simulink model "app_FaultMgr"  (R2016b)
settings: Solver=FixedStepDiscrete  StartTime=0.0  StopTime=10.0  FixedStep=0.001  RelTol=1e-3  EnableMultiTasking=on
PreLoadFcn:
  | try
  |    tapas_types('load');
  | catch
  |   disp('TAPAS WARNING: Tapas Types could not be loaded ...');
  | end
  | 
  | try
  |   app_types('load');
  | catch
  |   currdir =pwd;
  |   try
  |     cd('..\app_types\');
  |     app_types('load');
  |     cd(currdir);
  |   catch
  |     try
  |        cd('..\..\app_types\');
  |        app_types('load');
  |        cd(currdir);
  |     catch
  |        cd(currdir);
  |        disp('TAPAS WARNING: Application Types could not be loaded ...');
  |     end
  |   end
  |   try
  |       clear currdir;
  |   catch
  |      %Do nothing
  |   end
  | end
settings Model: Creator=kmansour  LastModifiedBy=Paul
settings DataIOCC: LimitDataPoints=on  SaveFormat=Array
settings OptimizationCC: LifeSpan=1
settings DebuggingCC: AllowSymbolicDim=off  SFUnexpectedBacktrackingDiag=warning  SFNoUnconditionalDefaultTransitionDiag=warning  SFExecutionAtInitializationDiag=none
settings HardwareCC: ProdBitPerPointer=32  ProdBitPerSizeT=32  ProdBitPerPtrDiffT=32  ProdLargestAtomicInteger=Long  ProdLargestAtomicFloat=Double  ProdWordSize=32  ProdHWDeviceType=Texas Instruments->TMS570 Cortex-R4
settings ModelReferenceCC: ModelReferenceNumInstancesAllowed=Single  PropagateSignalLabelsOutOfModel=off
settings RTWCC: SystemTargetFile=ert.tlc  GenCodeOnly=on  TemplateMakefile=ert_default_tmf  Description=Embedded Coder  GenerateReport=on  IncludeHyperlinkInReport=on  LaunchReport=on  GenerateTraceInfo=on  GenerateTraceReport=on  GenerateTraceReportSl=on  GenerateTraceReportSf=on  GenerateTraceReportEml=on
settings CodeAppCC: IgnoreCustomStorageClasses=off  MaxIdLength=63
settings ERTTargetCC: GenerateSampleERTMain=on  ERTSrcFileBannerTemplate=tapas_code_template.cgt  ERTHdrFileBannerTemplate=tapas_code_template.cgt  ERTDataSrcFileTemplate=tapas_code_template.cgt  ERTDataHdrFileTemplate=tapas_code_template.cgt  ERTCustomFileTemplate=example_file_process.tlc  ConvertIfToSwitch=off  SuppressUnreachableDefaultCases=off
settings ConfigComp: CovMetricSettings=dw  CovHtmlReporting=on  CovSaveCumulativeToWorkspaceVar=on  CovSaveSingleToWorkspaceVar=on  CovExternalEMLEnable=off

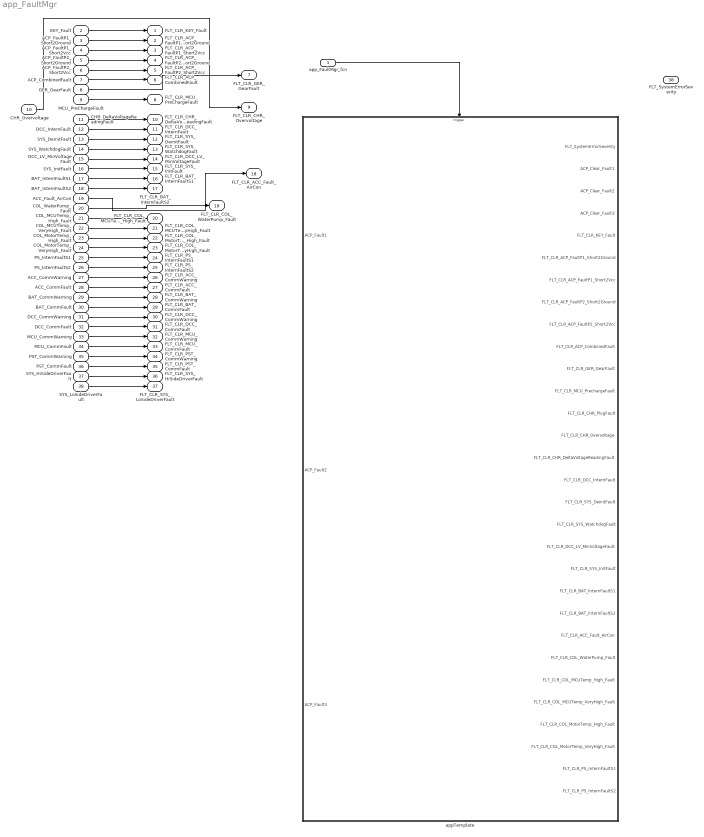
== system app_FaultMgr ==
  app_FaultMgr_fcn : Inport  SampleTime=1e-3  OutputFunctionCall=on
  KEY_Fault : Inport  Port=2
  ACP_FaultP1_Short2Ground : Inport  Port=3
  ACP_FaultP1_Short2Vcc : Inport  Port=4
  ACP_FaultP2_Short2Ground : Inport  Port=5
  ACP_FaultP2_Short2Vcc : Inport  Port=6
  ACP_CombinedFault : Inport  Port=7
  GER_GearFault : Inport  Port=8
  MCU_PreChargeFault : Inport  Port=9
  CHR_Overvoltage : Inport  Port=10
  CHR_DeltaVoltageReadingFault : Inport  Port=11
  DCC_InternFault : Inport  Port=12
  SYS_DeinitFault : Inport  Port=13
  SYS_WatchdogFault : Inport  Port=14
  DCC_LV_MinVoltageFault : Inport  Port=15
  SYS_InitFault : Inport  Port=16
  BAT_InternFaultS1 : Inport  Port=17
  BAT_InternFaultS2 : Inport  Port=18
  ACC_Fault_AirCon : Inport  Port=19
  COL_WaterPump_Fault : Inport  Port=20
  COL_MCUTemp_High_Fault : Inport  Port=21
  COL_MCUTemp_VeryHigh_Fault : Inport  Port=22
  COL_MotorTemp_High_Fault : Inport  Port=23
  COL_MotorTemp_VeryHigh_Fault : Inport  Port=24
  PS_InternFaultS1 : Inport  Port=25
  PS_InternFaultS2 : Inport  Port=26
  ACC_CommWarning : Inport  Port=27
  ACC_CommFault : Inport  Port=28
  BAT_CommWarning : Inport  Port=29
  BAT_CommFault : Inport  Port=30
  DCC_CommWarning : Inport  Port=31
  DCC_CommFault : Inport  Port=32
  MCU_CommWarning : Inport  Port=33
  MCU_CommFault : Inport  Port=34
  PST_CommWarning : Inport  Port=35
  PST_CommFault : Inport  Port=36
  SYS_HiSideDriverFault : Inport  Port=37
  SYS_LoSideDriverFault : Inport  Port=38
  appTemplate : Subsystem
  FLT_CLR_KEY_Fault : Outport
  FLT_CLR_ACP_FaultP1_Short2Ground : Outport  Port=2
  FLT_CLR_ACP_FaultP1_Short2Vcc : Outport  Port=3
  FLT_CLR_ACP_FaultP2_Short2Ground : Outport  Port=4
  FLT_CLR_ACP_FaultP2_Short2Vcc : Outport  Port=5
  FLT_CLR_ACP_CombinedFault : Outport  Port=6
  FLT_CLR_GER_GearFault : Outport  Port=7
  FLT_CLR_MCU_PreChargeFault : Outport  Port=8
  FLT_CLR_CHR_Overvoltage : Outport  Port=9
  FLT_CLR_CHR_DeltaVoltageReadingFault : Outport  Port=10
  FLT_CLR_DCC_InternFault : Outport  Port=11
  FLT_CLR_SYS_DeinitFault : Outport  Port=12
  FLT_CLR_SYS_WatchdogFault : Outport  Port=13
  FLT_CLR_DCC_LV_MinVoltageFault : Outport  Port=14
  FLT_CLR_SYS_InitFault : Outport  Port=15
  FLT_CLR_BAT_InternFaultS1 : Outport  Port=16
  FLT_CLR_BAT_InternFaultS2 : Outport  Port=17
  FLT_CLR_ACC_Fault_AirCon : Outport  Port=18
  FLT_CLR_COL_WaterPump_Fault : Outport  Port=19
  FLT_CLR_COL_MCUTemp_High_Fault : Outport  Port=20
  FLT_CLR_COL_MCUTemp_VeryHigh_Fault : Outport  Port=21
  FLT_CLR_COL_MotorTemp_High_Fault : Outport  Port=22
  FLT_CLR_COL_MotorTemp_VeryHigh_Fault : Outport  Port=23
  FLT_CLR_PS_InternFaultS1 : Outport  Port=24
  FLT_CLR_PS_InternFaultS2 : Outport  Port=25
  FLT_CLR_ACC_CommWarning : Outport  Port=26
  FLT_CLR_ACC_CommFault : Outport  Port=27
  FLT_CLR_BAT_CommWarning : Outport  Port=28
  FLT_CLR_BAT_CommFault : Outport  Port=29
  FLT_CLR_DCC_CommWarning : Outport  Port=30
  FLT_CLR_DCC_CommFault : Outport  Port=31
  FLT_CLR_MCU_CommWarning : Outport  Port=32
  FLT_CLR_MCU_CommFault : Outport  Port=33
  FLT_CLR_PST_CommWarning : Outport  Port=34
  FLT_CLR_PST_CommFault : Outport  Port=35
  FLT_CLR_SYS_HiSideDriverFault : Outport  Port=36
  FLT_CLR_SYS_LoSideDriverFault : Outport  Port=37
  FLT_SystemErrorSeverity : Outport  Port=38
  wires:
  app_FaultMgr_fcn/1 -> appTemplate/Trigger
  KEY_Fault/1 -> FLT_CLR_KEY_Fault/1
  ACP_FaultP1_Short2Ground/1 -> FLT_CLR_ACP_FaultP1_Short2Ground/1
  ACP_FaultP1_Short2Vcc/1 -> FLT_CLR_ACP_FaultP1_Short2Vcc/1
  ACP_FaultP2_Short2Ground/1 -> FLT_CLR_ACP_FaultP2_Short2Ground/1
  ACP_FaultP2_Short2Vcc/1 -> FLT_CLR_ACP_FaultP2_Short2Vcc/1
  ACP_CombinedFault/1 -> FLT_CLR_ACP_CombinedFault/1
  GER_GearFault/1 -> FLT_CLR_GER_GearFault/1
  MCU_PreChargeFault/1 -> FLT_CLR_MCU_PreChargeFault/1
  CHR_Overvoltage/1 -> FLT_CLR_CHR_Overvoltage/1
  CHR_DeltaVoltageReadingFault/1 -> FLT_CLR_CHR_DeltaVoltageReadingFault/1
  DCC_InternFault/1 -> FLT_CLR_DCC_InternFault/1
  SYS_DeinitFault/1 -> FLT_CLR_SYS_DeinitFault/1
  SYS_WatchdogFault/1 -> FLT_CLR_SYS_WatchdogFault/1
  DCC_LV_MinVoltageFault/1 -> FLT_CLR_DCC_LV_MinVoltageFault/1
  SYS_InitFault/1 -> FLT_CLR_SYS_InitFault/1
  BAT_InternFaultS1/1 -> FLT_CLR_BAT_InternFaultS1/1
  BAT_InternFaultS2/1 -> FLT_CLR_BAT_InternFaultS2/1
  ACC_Fault_AirCon/1 -> FLT_CLR_ACC_Fault_AirCon/1
  COL_WaterPump_Fault/1 -> FLT_CLR_COL_WaterPump_Fault/1
  COL_MCUTemp_High_Fault/1 -> FLT_CLR_COL_MCUTemp_High_Fault/1
  COL_MCUTemp_VeryHigh_Fault/1 -> FLT_CLR_COL_MCUTemp_VeryHigh_Fault/1
  COL_MotorTemp_High_Fault/1 -> FLT_CLR_COL_MotorTemp_High_Fault/1
  COL_MotorTemp_VeryHigh_Fault/1 -> FLT_CLR_COL_MotorTemp_VeryHigh_Fault/1
  PS_InternFaultS1/1 -> FLT_CLR_PS_InternFaultS1/1
  PS_InternFaultS2/1 -> FLT_CLR_PS_InternFaultS2/1
  ACC_CommWarning/1 -> FLT_CLR_ACC_CommWarning/1
  ACC_CommFault/1 -> FLT_CLR_ACC_CommFault/1
  BAT_CommWarning/1 -> FLT_CLR_BAT_CommWarning/1
  BAT_CommFault/1 -> FLT_CLR_BAT_CommFault/1
  DCC_CommWarning/1 -> FLT_CLR_DCC_CommWarning/1
  DCC_CommFault/1 -> FLT_CLR_DCC_CommFault/1
  MCU_CommWarning/1 -> FLT_CLR_MCU_CommWarning/1
  MCU_CommFault/1 -> FLT_CLR_MCU_CommFault/1
  PST_CommWarning/1 -> FLT_CLR_PST_CommWarning/1
  PST_CommFault/1 -> FLT_CLR_PST_CommFault/1
  SYS_HiSideDriverFault/1 -> FLT_CLR_SYS_HiSideDriverFault/1
  SYS_LoSideDriverFault/1 -> FLT_CLR_SYS_LoSideDriverFault/1

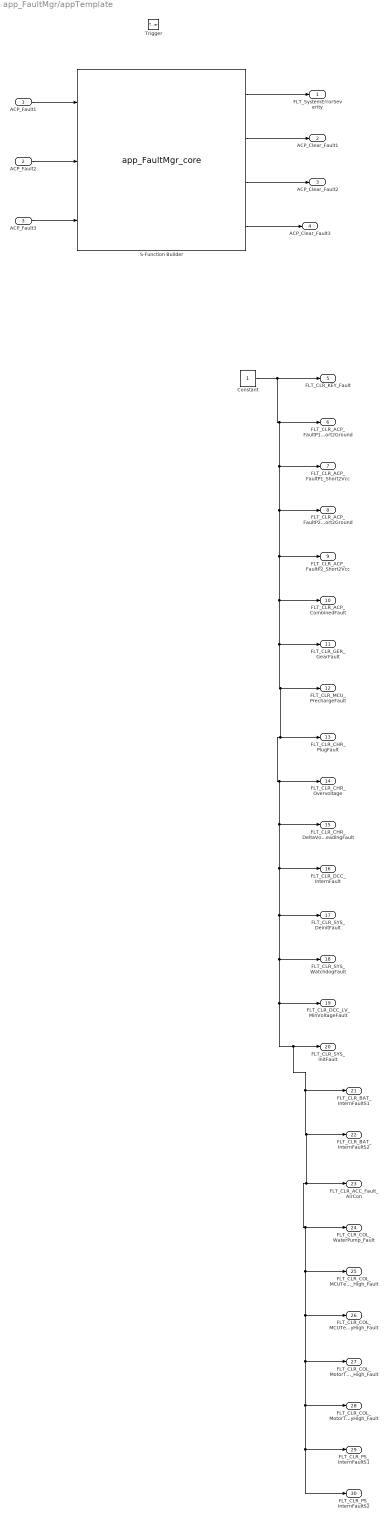
== system app_FaultMgr/appTemplate ==
  ACP_Fault1 : Inport
  ACP_Fault2 : Inport  Port=2
  ACP_Fault3 : Inport  Port=3
  Trigger : TriggerPort  TriggerType=function-call  VariantControl=Variant  SampleTimeType=periodic  SampleTime=-1  PortDimensions=1
  Constant : Constant
  S-Function Builder : S-Function  InitFcn=try, set_param(gcb,'FunctionName','app_FaultMgr_core'), end  FunctionName=app_FaultMgr_core  SFunctionModules=app_FaultMgr_core_wrapper rte stub app_FaultMgr app_FaultMgr_cfg  SFunctionDeploymentMode=off  EnableBusSupport=off  mask(S-Function Builder){}
      mask help: Simulink:masks:SFunctionBuilder_MD
      mask init:
      | val = [[.9  0.75 0.75 1 1 .9 .9 1]',[1 1 0.75 0.75 .9 .9 1 .9]'];try , sys = get_param(gcb,'SfunBuilderFcnName');if isempty(sys), sys = get_param(gcb,'FunctionName'); end,catch, sys = get_param(gcb,'FunctionName'); end
      settings: CopyFcn=set_param(gcbh,'LinkStatus','none')  PreSaveFcn=try, set_param(gcb,'FunctionName','app_FaultMgr_core'), end  OpenFcn=sfunctionwizard(gcbh)
      mask Display: plot(val(:,1),val(:,2)),disp(sys), port_label('input',1,'ACP_Fault1'), port_label('input',2,'ACP_Fault2'), port_label('input',3,'ACP_Fault3'), port_label('output',1,'FLT_SystemErrorSeverity'), port_label('output',2,'ACP_Clear_Fault1'), port_label('output',3,'ACP_Clear_Fault2'), port_label('output',4,'ACP_Clear_Fault3')
  FLT_SystemErrorSeverity : Outport
  ACP_Clear_Fault1 : Outport  Port=2
  ACP_Clear_Fault2 : Outport  Port=3
  ACP_Clear_Fault3 : Outport  Port=4
  FLT_CLR_KEY_Fault : Outport  Port=5
  FLT_CLR_ACP_FaultP1_Short2Ground : Outport  Port=6
  FLT_CLR_ACP_FaultP1_Short2Vcc : Outport  Port=7
  FLT_CLR_ACP_FaultP2_Short2Ground : Outport  Port=8
  FLT_CLR_ACP_FaultP2_Short2Vcc : Outport  Port=9
  FLT_CLR_ACP_CombinedFault : Outport  Port=10
  FLT_CLR_GER_GearFault : Outport  Port=11
  FLT_CLR_MCU_PrechargeFault : Outport  Port=12
  FLT_CLR_CHR_PlugFault : Outport  Port=13
  FLT_CLR_CHR_Overvoltage : Outport  Port=14
  FLT_CLR_CHR_DeltaVoltageReadingFault : Outport  Port=15
  FLT_CLR_DCC_InternFault : Outport  Port=16
  FLT_CLR_SYS_DeinitFault : Outport  Port=17
  FLT_CLR_SYS_WatchdogFault : Outport  Port=18
  FLT_CLR_DCC_LV_MinVoltageFault : Outport  Port=19
  FLT_CLR_SYS_InitFault : Outport  Port=20
  FLT_CLR_BAT_InternFaultS1 : Outport  Port=21
  FLT_CLR_BAT_InternFaultS2 : Outport  Port=22
  FLT_CLR_ACC_Fault_AirCon : Outport  Port=23
  FLT_CLR_COL_WaterPump_Fault : Outport  Port=24
  FLT_CLR_COL_MCUTemp_High_Fault : Outport  Port=25
  FLT_CLR_COL_MCUTemp_VeryHigh_Fault : Outport  Port=26
  FLT_CLR_COL_MotorTemp_High_Fault : Outport  Port=27
  FLT_CLR_COL_MotorTemp_VeryHigh_Fault : Outport  Port=28
  FLT_CLR_PS_InternFaultS1 : Outport  Port=29
  FLT_CLR_PS_InternFaultS2 : Outport  Port=30
  wires:
  S-Function Builder/1 -> FLT_SystemErrorSeverity/1
  S-Function Builder/2 -> ACP_Clear_Fault1/1
  S-Function Builder/3 -> ACP_Clear_Fault2/1
  S-Function Builder/4 -> ACP_Clear_Fault3/1
  ACP_Fault1/1 -> S-Function Builder/1
  ACP_Fault2/1 -> S-Function Builder/2
  ACP_Fault3/1 -> S-Function Builder/3
  Constant/1 -> FLT_CLR_GER_GearFault/1, FLT_CLR_CHR_Overvoltage/1, FLT_CLR_CHR_DeltaVoltageReadingFault/1, FLT_CLR_DCC_InternFault/1, FLT_CLR_SYS_DeinitFault/1, FLT_CLR_SYS_WatchdogFault/1, FLT_CLR_SYS_InitFault/1, FLT_CLR_BAT_InternFaultS2/1, FLT_CLR_ACC_Fault_AirCon/1, FLT_CLR_PS_InternFaultS1/1, FLT_CLR_PS_InternFaultS2/1, FLT_CLR_COL_MotorTemp_VeryHigh_Fault/1, FLT_CLR_COL_MotorTemp_High_Fault/1, FLT_CLR_COL_MCUTemp_VeryHigh_Fault/1, FLT_CLR_COL_MCUTemp_High_Fault/1, FLT_CLR_COL_WaterPump_Fault/1, FLT_CLR_BAT_InternFaultS1/1, FLT_CLR_DCC_LV_MinVoltageFault/1, FLT_CLR_CHR_PlugFault/1, FLT_CLR_MCU_PrechargeFault/1, FLT_CLR_ACP_CombinedFault/1, FLT_CLR_ACP_FaultP2_Short2Vcc/1, FLT_CLR_ACP_FaultP2_Short2Ground/1, FLT_CLR_ACP_FaultP1_Short2Vcc/1, FLT_CLR_ACP_FaultP1_Short2Ground/1, FLT_CLR_KEY_Fault/1
